simulink model "model"  (R2020b)
settings: Solver=VariableStepAuto  StartTime=0.0  StopTime=1  FixedStep=Ts  RelTol=1e-3
model workspace (MAT data in the model file):
  J = Simulink.Parameter
  J.Value = 3.2284e-06
  J.DataType = 'auto'
  J.Dimensions = [1 1]
  Ke = Simulink.Parameter
  Ke.Value = 0.0274
  Ke.DataType = 'auto'
  Ke.Dimensions = [1 1]
  Kt = Simulink.Parameter
  Kt.Value = 0.0274
  Kt.DataType = 'auto'
  Kt.Dimensions = [1 1]
  L = Simulink.Parameter
  L.Value = 2.75e-06
  L.DataType = 'auto'
  L.Dimensions = [1 1]
  R = Simulink.Parameter
  R.Value = 4
  R.DataType = 'auto'
  R.Dimensions = [1 1]
  Ts = Simulink.Parameter
  Ts.Value = 0.01
  Ts.DataType = 'auto'
  Ts.Dimensions = [1 1]
  b = Simulink.Parameter
  b.Value = 3.5077e-06
  b.DataType = 'auto'
  b.Dimensions = [1 1]
settings Model: OrderedModelArguments=off  Creator=Lenovo  LastModifiedBy=HP

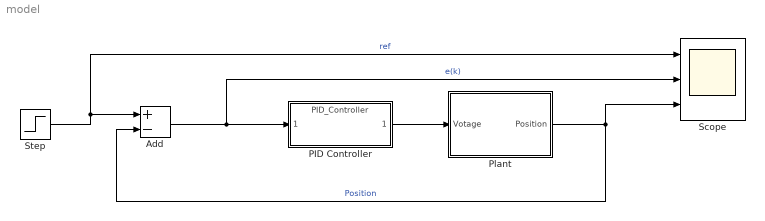
== system model ==
  Add : Sum  Inputs=+-
  PID Controller : ModelReference  ModelNameDialog=PID_Controller  SimulationMode=Normal  ModelReferenceVersion=1.47  mask{Kp=881695.95, Ki=39026037545.99, Kd=49.11, N=0}
  Plant : Subsystem
  Scope : Scope  NumInputPorts=3
  Step : Step  Time=0  SampleTime=0
  wires:
  Plant/1(Position) -> Add/2, Scope/3  "Position"
  Step/1 -> Add/1, Scope/1  "ref"
  Add/1 -> PID Controller/1, Scope/2  "e(k)"
  PID Controller/1 -> Plant/1(Votage)

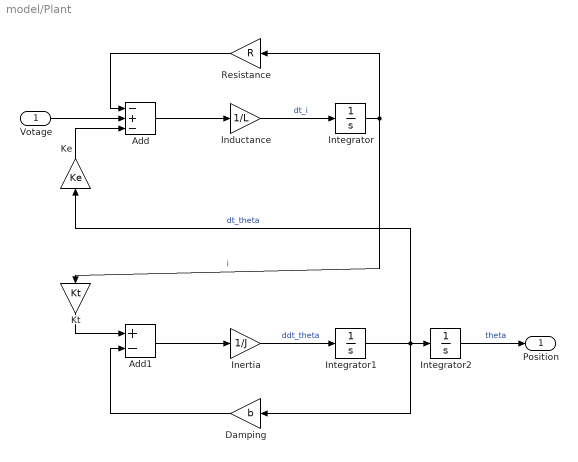
== system model/Plant ==
  Votage : Inport
  Add : Sum  Inputs=-+-
  Add1 : Sum  Inputs=+-
  Damping : Gain  Gain=b
  Inductance : Gain  Gain=1/L
  Inertia : Gain  Gain=1/J
  Integrator : Integrator
  Integrator1 : Integrator
  Integrator2 : Integrator
  Ke : Gain  Gain=Ke
  Kt : Gain  Gain=Kt
  Resistance : Gain  Gain=R
  Position : Outport
  wires:
  Add/1 -> Inductance/1
  Inductance/1 -> Integrator/1  "dt_i"
  Integrator/1 -> Resistance/1, Kt/1  "i"
  Resistance/1 -> Add/1
  Add1/1 -> Inertia/1
  Inertia/1 -> Integrator1/1  "ddt_theta"
  Integrator1/1 -> Ke/1, Integrator2/1, Damping/1  "dt_theta"
  Damping/1 -> Add1/2
  Ke/1 -> Add/3
  Votage/1 -> Add/2
  Kt/1 -> Add1/1
  Integrator2/1 -> Position/1  "theta"
